simulink model "mpc_pathFollowingMod"  (R2024a)
settings: Solver=VariableStepAuto  StartTime=0.0  StopTime=10.0  RelTol=1e-3
PreLoadFcn:
  | load('pathFollowingUtil\pfcsubsystem_data.mat');
  | load('pathFollowingUtil\mpc_base.mat');
values from neighbouring files (symbols this model uses):
  Cf = evalin('base','Cf')    [helperSLTrajectoryFollowerWithRRScenarioSetup.m]
  Cr = evalin('base','Cr')    [helperSLTrajectoryFollowerWithRRScenarioSetup.m]
  Iz = evalin('base','Iz')    [helperSLTrajectoryFollowerWithRRScenarioSetup.m]
  lf = evalin('base','lf')    [helperSLTrajectoryFollowerWithRRScenarioSetup.m]
  lr = evalin('base','lr')    [helperSLTrajectoryFollowerWithRRScenarioSetup.m]
  m = worldActors(idx).actor_runtime.pose.matrix    [helperSLTrajectoryFollowerWithRRScenarioSetup.m]
  numReferencePose = 1    [HelperReferencePoseOnPath.m]
  pfcsubsystem_data =     [pfcsubsystem_data.mat]
undefined symbols (not defined in the file or in its folder): control_timeStep, DefaultSpacing, E_mpc, F_mpc, hasLag, InitialLongVel, NumEgoStates, sizeExNumSS, tau, tau2
libraries: mpcsigdimcheck_private x19, mpclib x3, simulink x2, sharedTrackingLibrary x1
(part 1 of 2)
settings Model: Creator=nobuakif  LastModifiedBy=fukuchi
settings DebuggingCC: UnderSpecifiedDimensionMsg=warning

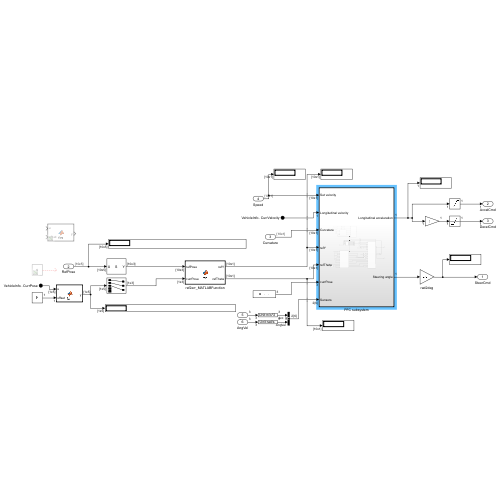
[thumbnail: Simulink's stored preview of the top-level diagram]
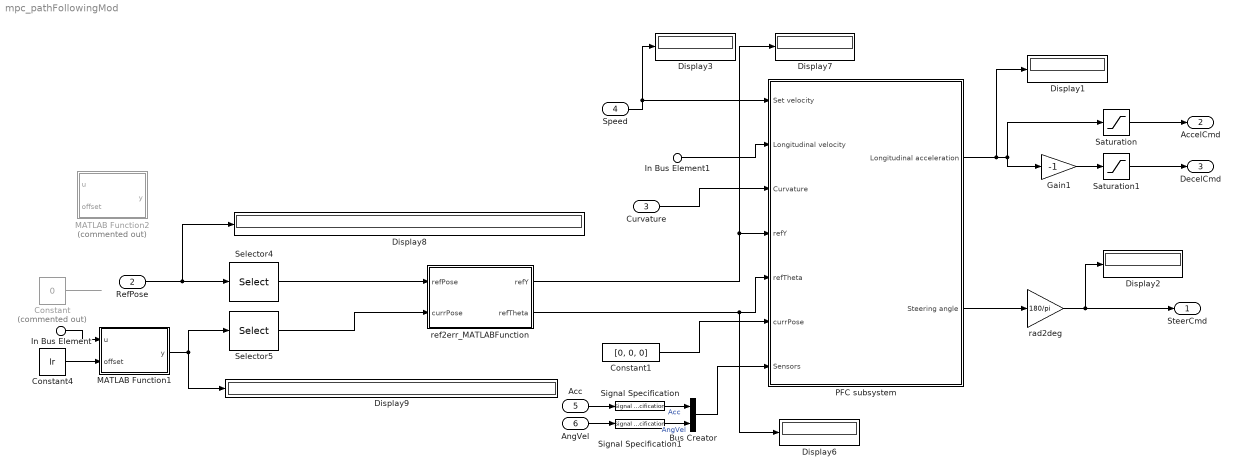
== system mpc_pathFollowingMod ==
  In Bus Element : Inport  PortName=VehicleInfo  Element=CurrPose
  In Bus Element1 : Inport  PortName=VehicleInfo  Element=CurrVelocity
  RefPose : Inport  Port=2  PortDimensions=[numReferencePose, 5]
  Curvature : Inport  Port=3  PortDimensions=[numReferencePose, 1]
  Speed : Inport  Port=4  PortDimensions=[numReferencePose, 1]
  Acc : Inport  Port=5  PortDimensions=3
  AngVel : Inport  Port=6  PortDimensions=3
  Bus Creator : BusCreator  Inputs=2
  Constant : Constant  Commented=on  Value=0
  Constant1 : Constant  Value=[0, 0, 0]
  Constant4 : Constant  Value=lr
  Display{1..3,6..9} (7 alike) : Display
  Gain1 : Gain  Gain=-1
  MATLAB Function1 : MATLAB Function  TreatAsAtomicUnit=on
  MATLAB Function2 : MATLAB Function  Commented=on  TreatAsAtomicUnit=on
  PFC subsystem : Subsystem  TreatAsAtomicUnit=on  VariantControl=Variant2
      settings: LibrarySourceBlock=mpclib/Automated Driving/Path Following Control System  RTWFileNameOpts=Use function name
  Saturation : Saturate  UpperLimit=inf  LowerLimit=0
  Saturation1 : Saturate  UpperLimit=inf  LowerLimit=0
  Selector4 : Selector  NumberOfDimensions=2  InputPortWidth=5  IndexOptions=Select all,Index vector (dialog)  Indices=[1:3],[1:3]  OutputSizes=1,1
  Selector5 : Selector  InputPortWidth=5  IndexOptions=Index vector (dialog)  Indices=[1:3]  OutputSizes=1
  Signal Specification : SignalSpecification  Unit=m/s^2
  Signal Specification1 : SignalSpecification  Unit=rad/s
  rad2deg : Gain  Gain=180/pi
  ref2err_MATLABFunction : MATLAB Function  TreatAsAtomicUnit=on
  SteerCmd : Outport
  AccelCmd : Outport  Port=2
  DecelCmd : Outport  Port=3
  wires:
  rad2deg/1 -> SteerCmd/1, Display2/1
  Saturation/1 -> AccelCmd/1
  Selector4/1 -> ref2err_MATLABFunction/1(refPose)
  Saturation1/1 -> DecelCmd/1
  MATLAB Function1/1(y) -> Selector5/1, Display9/1
  Selector5/1 -> ref2err_MATLABFunction/2(currPose)
  Constant/1 -> ?
  PFC subsystem/1(Longitudinal acceleration) -> Display1/1, Saturation/1, Gain1/1
  Constant4/1 -> MATLAB Function1/2(offset)
  In Bus Element/1 -> MATLAB Function1/1(u)
  RefPose/1 -> Display8/1, Selector4/1
  PFC subsystem/2(Steering angle) -> rad2deg/1
  In Bus Element1/1 -> PFC subsystem/2(Longitudinal velocity)
  Curvature/1 -> PFC subsystem/3(Curvature)
  ref2err_MATLABFunction/1(refY) -> PFC subsystem/4(refY), Display7/1
  ref2err_MATLABFunction/2(refTheta) -> Display6/1, PFC subsystem/5(refTheta)
  Speed/1 -> Display3/1, PFC subsystem/1(Set velocity)
  Gain1/1 -> Saturation1/1
  Constant1/1 -> PFC subsystem/6(currPose)
  Acc/1 -> Signal Specification/1
  Bus Creator/1 -> PFC subsystem/7(Sensors)
  AngVel/1 -> Signal Specification1/1
  Signal Specification/1 -> Bus Creator/1  "Acc"
  Signal Specification1/1 -> Bus Creator/2  "AngVel"

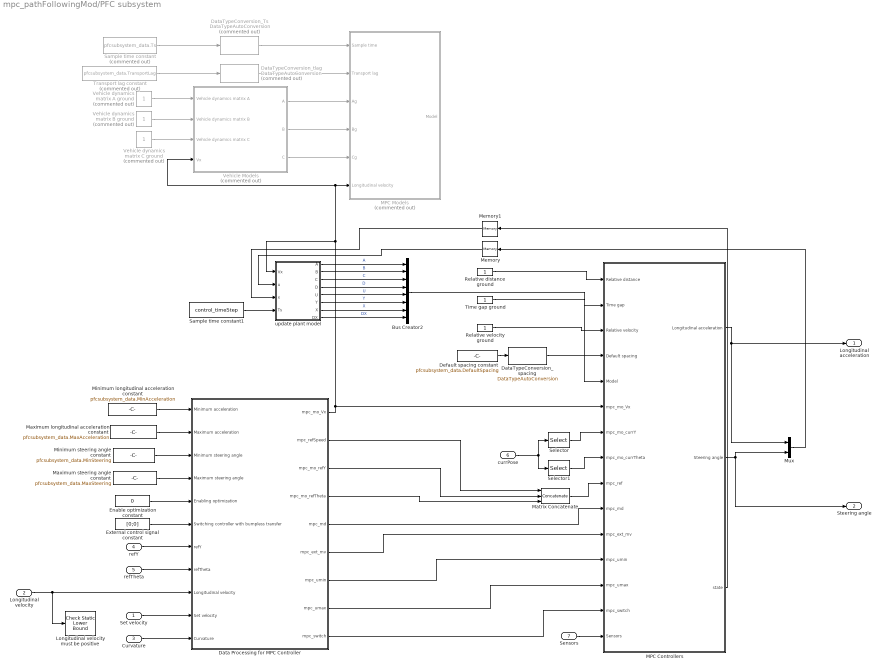
== system mpc_pathFollowingMod/PFC subsystem ==
  Set velocity : Inport
  Longitudinal velocity : Inport  Port=2
  Curvature : Inport  Port=3
  refY : Inport  Port=4
  refTheta : Inport  Port=5
  currPose : Inport  Port=6
  Sensors : Inport  Port=7
  Bus Creator2 : BusCreator  Inputs=8
  Data Processing for MPC Controller : Subsystem
  DataTypeConversion_Ts : mpcsigdimcheck_private/DataTypeAutoConversion  Commented=on  datatypestr=pfcsubsystem_data.DataType
  DataTypeConversion_spacing : mpcsigdimcheck_private/DataTypeAutoConversion  datatypestr=pfcsubsystem_data.DataType
  DataTypeConversion_tlag : mpcsigdimcheck_private/DataTypeAutoConversion  Commented=on  datatypestr=pfcsubsystem_data.DataType
  Default spacing constant : Constant  Value=pfcsubsystem_data.DefaultSpacing  OutDataTypeStr=pfcsubsystem_data.DataType
  Enable optimization constant : Constant  Value=0  OutDataTypeStr=pfcsubsystem_data.DataType
  External control signal constant : Constant  Value=[0;0]  VectorParams1D=off  OutDataTypeStr=pfcsubsystem_data.DataType
  Longitudinal velocity must be positive : simulink/Model Verification/Check Static  Lower Bound  Description=0 < u  min=0  min_included=off  enabled=on  stopWhenAssertionFail=on  export=off  icon=graphic
  MPC Controllers : Subsystem  Variant=on  VariantControlMode=label  VariantControl=Variant1  LabelModeActiveChoice=pathFollowingNoSpacingCtrl
  MPC Models : Subsystem  Commented=on  Variant=on  VariantControlMode=label  VariantControl=Variant1  LabelModeActiveChoice=pathFollowingNoSpacingCtrl
  Matrix Concatenate : Concatenate  NumInputs=3  Mode=Multidimensional array  ConcatenateDimension=2
  Maximum longitudinal acceleration constant : Constant  Value=pfcsubsystem_data.MaxAcceleration  OutDataTypeStr=pfcsubsystem_data.DataType
  Maximum steering angle constant : Constant  Value=pfcsubsystem_data.MaxSteering  OutDataTypeStr=pfcsubsystem_data.DataType
  Memory : Memory
  Memory1 : Memory
  Minimum longitudinal acceleration constant : Constant  Value=pfcsubsystem_data.MinAcceleration  OutDataTypeStr=pfcsubsystem_data.DataType
  Minimum steering angle constant : Constant  Value=pfcsubsystem_data.MinSteering  OutDataTypeStr=pfcsubsystem_data.DataType
  Mux : Mux  Inputs=2
  Relative distance ground : Constant  OutDataTypeStr=pfcsubsystem_data.DataType
  Relative velocity ground : Constant  OutDataTypeStr=pfcsubsystem_data.DataType
  Sample time constant : Constant  Commented=on  Value=pfcsubsystem_data.Ts  OutDataTypeStr=pfcsubsystem_data.DataType
  Sample time constant1 : Constant  Value=control_timeStep  OutDataTypeStr=pfcsubsystem_data.DataType
  Selector : Selector  InputPortWidth=3  IndexOptions=Index vector (dialog)  Indices=2  OutputSizes=1
  Selector1 : Selector  InputPortWidth=3  IndexOptions=Index vector (dialog)  Indices=3  OutputSizes=1
  Time gap ground : Constant  OutDataTypeStr=pfcsubsystem_data.DataType
  Transport lag constant : Constant  Commented=on  Value=pfcsubsystem_data.TransportLag  OutDataTypeStr=pfcsubsystem_data.DataType
  Vehicle Models : Subsystem  Commented=on  Variant=on  VariantControlMode=label  VariantControl=Variant1  LabelModeActiveChoice=useVehicleParameters
  Vehicle dynamics matrix A ground : Constant  Commented=on  OutDataTypeStr=pfcsubsystem_data.DataType
  Vehicle dynamics matrix B ground : Constant  Commented=on  OutDataTypeStr=pfcsubsystem_data.DataType
  Vehicle dynamics matrix C ground : Constant  Commented=on  OutDataTypeStr=pfcsubsystem_data.DataType
  update plant model : MATLAB Function  TreatAsAtomicUnit=on
  Longitudinal acceleration : Outport  PortDimensions=1  VectorParamsAs1DForOutWhenUnconnected=off
  Steering angle : Outport  Port=2  VectorParamsAs1DForOutWhenUnconnected=off
  wires:
  Relative velocity ground/1 -> MPC Controllers/3("Relative velocity ")
  Relative distance ground/1 -> MPC Controllers/1("Relative distance ")
  Time gap ground/1 -> MPC Controllers/2("Time gap ")
  MPC Controllers/1(" Longitudinal acceleration") -> Longitudinal acceleration/1, Mux/1
  Default spacing constant/1 -> DataTypeConversion_spacing/1
  Data Processing for MPC Controller/9(mpc_switch) -> MPC Controllers/14("mpc_switch ")
  Bus Creator2/1 -> MPC Controllers/5("Model ")
  Data Processing for MPC Controller/8(mpc_umax) -> MPC Controllers/13("mpc_umax ")
  Data Processing for MPC Controller/1(mpc_mo_Vx) -> update plant model/1(Vx), MPC Models/6("Longitudinal velocity "), Vehicle Models/4("Vx "), MPC Controllers/6("mpc_mo_Vx ")
  Data Processing for MPC Controller/5(mpc_md) -> MPC Controllers/10("mpc_md ")
  Data Processing for MPC Controller/4(mpc_mo_refTheta) -> Matrix Concatenate/3
  Data Processing for MPC Controller/2(mpc_refSpeed) -> Matrix Concatenate/1
  Longitudinal velocity/1 -> Data Processing for MPC Controller/9(Longitudinal velocity), Longitudinal velocity must be positive/1
  Data Processing for MPC Controller/3(mpc_mo_refY) -> Matrix Concatenate/2
  Data Processing for MPC Controller/6(mpc_ext_mv) -> MPC Controllers/11("mpc_ext_mv ")
  Data Processing for MPC Controller/7(mpc_umin) -> MPC Controllers/12("mpc_umin ")
  Curvature/1 -> Data Processing for MPC Controller/11(Curvature)
  Set velocity/1 -> Data Processing for MPC Controller/10(Set velocity)
  refY/1 -> Data Processing for MPC Controller/7(refY)
  refTheta/1 -> Data Processing for MPC Controller/8(refTheta)
  Maximum longitudinal acceleration constant/1 -> Data Processing for MPC Controller/2(Maximum acceleration)
  Maximum steering angle constant/1 -> Data Processing for MPC Controller/4(Maximum steering angle)
  Enable optimization constant/1 -> Data Processing for MPC Controller/5(Enabling optimization)
  External control signal constant/1 -> Data Processing for MPC Controller/6(Switching controller with bumpless transfer)
  Minimum longitudinal acceleration constant/1 -> Data Processing for MPC Controller/1(Minimum acceleration)
  Minimum steering angle constant/1 -> Data Processing for MPC Controller/3(Minimum steering angle)
  Vehicle Models/1(" A") -> MPC Models/3(Ag)
  Vehicle Models/2(" B") -> MPC Models/4(Bg)
  Vehicle Models/3(" C") -> MPC Models/5(Cg)
  Transport lag constant/1 -> DataTypeConversion_tlag/1
  Sample time constant/1 -> DataTypeConversion_Ts/1
  Vehicle dynamics matrix A ground/1 -> Vehicle Models/1(Vehicle dynamics matrix A)
  Vehicle dynamics matrix C ground/1 -> Vehicle Models/3(Vehicle dynamics matrix C)
  Vehicle dynamics matrix B ground/1 -> Vehicle Models/2(Vehicle dynamics matrix B)
  DataTypeConversion_Ts/1 -> MPC Models/1(Sample time)
  DataTypeConversion_tlag/1 -> MPC Models/2(Transport lag)
  DataTypeConversion_spacing/1 -> MPC Controllers/4("Default spacing ")
  Sample time constant1/1 -> update plant model/4(Ts)
  update plant model/1(A) -> Bus Creator2/1  "A"
  update plant model/2(B) -> Bus Creator2/2  "B"
  update plant model/3(C) -> Bus Creator2/3  "C"
  update plant model/4(D) -> Bus Creator2/4  "D"
  update plant model/5(U) -> Bus Creator2/5  "U"
  update plant model/6(Y) -> Bus Creator2/6  "Y"
  update plant model/7(X) -> Bus Creator2/7  "X"
  update plant model/8(DX) -> Bus Creator2/8  "DX"
  Mux/1 -> Memory/1
  MPC Controllers/3(state) -> Memory1/1
  Memory/1 -> update plant model/2(u)
  Matrix Concatenate/1 -> MPC Controllers/9("mpc_ref ")
  Selector/1 -> MPC Controllers/7(mpc_mo_currY)
  Selector1/1 -> MPC Controllers/8(mpc_mo_currTheta)
  currPose/1 -> Selector1/1, Selector/1
  Memory1/1 -> update plant model/3(x)
  MPC Controllers/2("  Steering angle") -> Mux/2, Steering angle/1
  Sensors/1 -> MPC Controllers/15(Sensors)

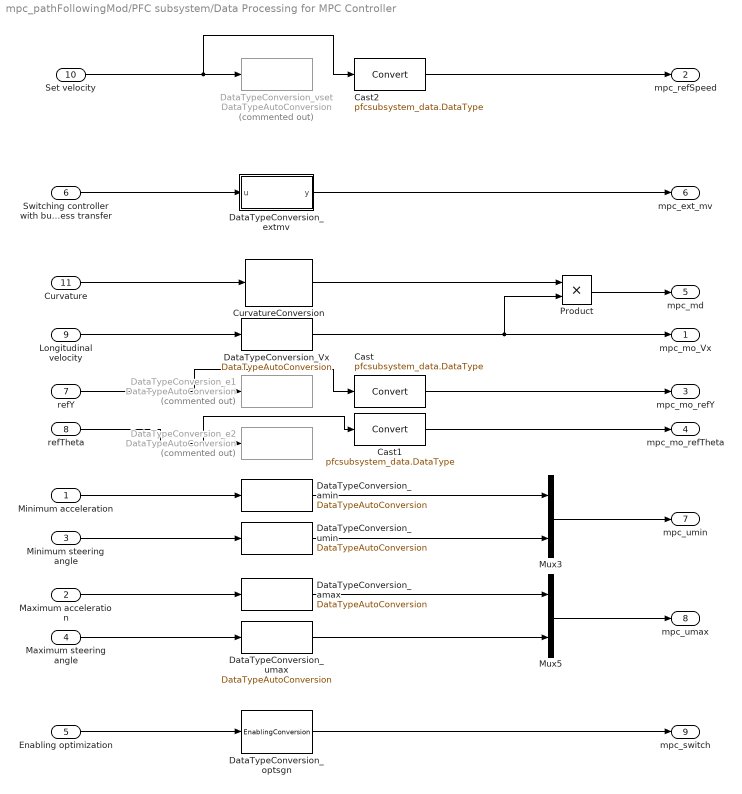
== system mpc_pathFollowingMod/PFC subsystem/Data Processing for MPC Controller ==
  Minimum acceleration : Inport
  Maximum acceleration : Inport  Port=2
  Minimum steering angle : Inport  Port=3
  Maximum steering angle : Inport  Port=4
  Enabling optimization : Inport  Port=5
  Switching controller with bumpless transfer : Inport  Port=6
  refY : Inport  Port=7
  refTheta : Inport  Port=8
  Longitudinal velocity : Inport  Port=9
  Set velocity : Inport  Port=10
  Curvature : Inport  Port=11
  Cast : DataTypeConversion  OutDataTypeStr=pfcsubsystem_data.DataType  SaturateOnIntegerOverflow=off  RndMeth=Floor
  Cast1 : DataTypeConversion  OutDataTypeStr=pfcsubsystem_data.DataType  SaturateOnIntegerOverflow=off  RndMeth=Floor
  Cast2 : DataTypeConversion  OutDataTypeStr=pfcsubsystem_data.DataType  SaturateOnIntegerOverflow=off  RndMeth=Floor
  CurvatureConversion : mpcsigdimcheck_private/CurvatureConversion  datatypestr=pfcsubsystem_data.DataType  p=pfcsubsystem_data.Controller.PredictionHorizon
  DataTypeConversion_Vx : mpcsigdimcheck_private/DataTypeAutoConversion  datatypestr=pfcsubsystem_data.DataType
  DataTypeConversion_amax : mpcsigdimcheck_private/DataTypeAutoConversion  datatypestr=pfcsubsystem_data.DataType
  DataTypeConversion_amin : mpcsigdimcheck_private/DataTypeAutoConversion  datatypestr=pfcsubsystem_data.DataType
  DataTypeConversion_e1 : mpcsigdimcheck_private/DataTypeAutoConversion  Commented=on  datatypestr=pfcsubsystem_data.DataType
  DataTypeConversion_e2 : mpcsigdimcheck_private/DataTypeAutoConversion  Commented=on  datatypestr=pfcsubsystem_data.DataType
  DataTypeConversion_extmv : MATLAB Function  TreatAsAtomicUnit=on  mask(MPCDataTypeAutoConversion){datatypestr=pfcsubsystem_data.DataType}
      mask prompts: datatypestr "Data type"
      mask init:
      | isDouble = strcmp(datatypestr,'double');
  DataTypeConversion_optsgn : mpcsigdimcheck_private/EnablingConversion  SystemSampleTime=-1  VariantActivationTime=update diagram  AllowFlexibleInterface=on  Latency=0  AutoFrameSizeCalculation=off
  DataTypeConversion_umax : mpcsigdimcheck_private/DataTypeAutoConversion  datatypestr=pfcsubsystem_data.DataType
  DataTypeConversion_umin : mpcsigdimcheck_private/DataTypeAutoConversion  datatypestr=pfcsubsystem_data.DataType
  DataTypeConversion_vset : mpcsigdimcheck_private/DataTypeAutoConversion  Commented=on  datatypestr=pfcsubsystem_data.DataType
  Mux3 : Mux  Inputs=2
  Mux5 : Mux  Inputs=2
  Product : Product
  mpc_mo_Vx : Outport  VectorParamsAs1DForOutWhenUnconnected=off
  mpc_refSpeed : Outport  Port=2  VectorParamsAs1DForOutWhenUnconnected=off
  mpc_mo_refY : Outport  Port=3  VectorParamsAs1DForOutWhenUnconnected=off
  mpc_mo_refTheta : Outport  Port=4  VectorParamsAs1DForOutWhenUnconnected=off
  mpc_md : Outport  Port=5  VectorParamsAs1DForOutWhenUnconnected=off
  mpc_ext_mv : Outport  Port=6  VectorParamsAs1DForOutWhenUnconnected=off
  mpc_umin : Outport  Port=7  VectorParamsAs1DForOutWhenUnconnected=off
  mpc_umax : Outport  Port=8  VectorParamsAs1DForOutWhenUnconnected=off
  mpc_switch : Outport  Port=9  VectorParamsAs1DForOutWhenUnconnected=off
  wires:
  Longitudinal velocity/1 -> DataTypeConversion_Vx/1
  Curvature/1 -> CurvatureConversion/1
  Mux5/1 -> mpc_umax/1
  Maximum steering angle/1 -> DataTypeConversion_umax/1
  Minimum steering angle/1 -> DataTypeConversion_umin/1
  DataTypeConversion_amin/1 -> Mux3/1
  CurvatureConversion/1 -> Product/1
  Product/1 -> mpc_md/1
  refTheta/1 -> Cast1/1, DataTypeConversion_e2/1
  Maximum acceleration/1 -> DataTypeConversion_amax/1
  refY/1 -> Cast/1, DataTypeConversion_e1/1
  DataTypeConversion_umin/1 -> Mux3/2
  DataTypeConversion_amax/1 -> Mux5/1
  DataTypeConversion_Vx/1 -> mpc_mo_Vx/1, Product/2
  DataTypeConversion_umax/1 -> Mux5/2
  Minimum acceleration/1 -> DataTypeConversion_amin/1
  Switching controller with bumpless transfer/1 -> DataTypeConversion_extmv/1(u)
  DataTypeConversion_extmv/1(y) -> mpc_ext_mv/1
  Mux3/1 -> mpc_umin/1
  Set velocity/1 -> Cast2/1, DataTypeConversion_vset/1
  Cast/1 -> mpc_mo_refY/1
  Enabling optimization/1 -> DataTypeConversion_optsgn/1
  DataTypeConversion_optsgn/1 -> mpc_switch/1
  Cast1/1 -> mpc_mo_refTheta/1
  Cast2/1 -> mpc_refSpeed/1

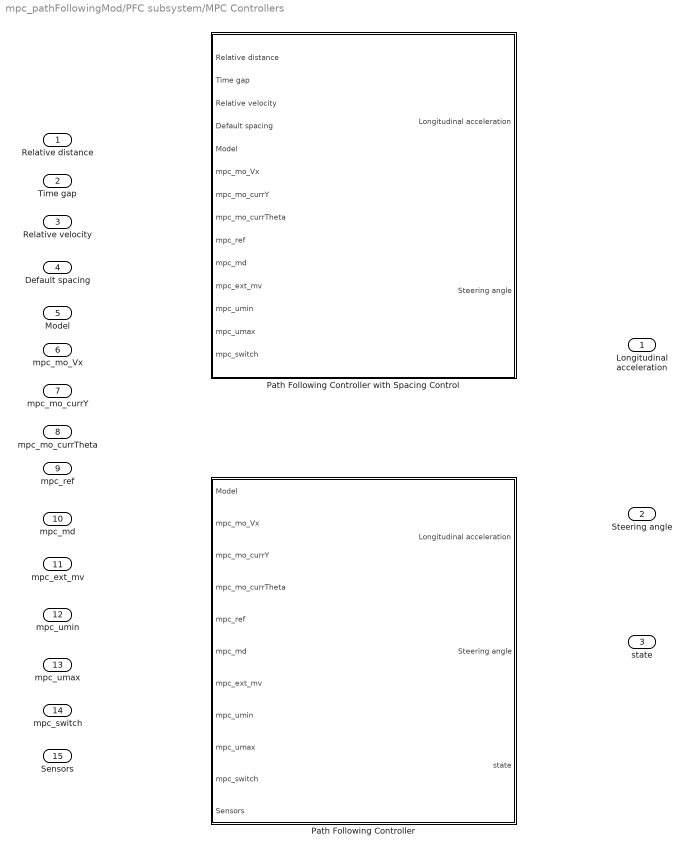
== system mpc_pathFollowingMod/PFC subsystem/MPC Controllers ==
  "Relative distance " : Inport
  "Time gap " : Inport  Port=2
  "Relative velocity " : Inport  Port=3
  "Default spacing " : Inport  Port=4
  "Model " : Inport  Port=5
  "mpc_mo_Vx " : Inport  Port=6
  mpc_mo_currY : Inport  Port=7
  mpc_mo_currTheta : Inport  Port=8
  "mpc_ref " : Inport  Port=9
  "mpc_md " : Inport  Port=10
  "mpc_ext_mv " : Inport  Port=11
  "mpc_umin " : Inport  Port=12
  "mpc_umax " : Inport  Port=13
  "mpc_switch " : Inport  Port=14
  Sensors : Inport  Port=15
  Path Following Controller : Subsystem  VariantControl=pathFollowingNoSpacingCtrl
  Path Following Controller with Spacing Control : Subsystem  VariantControl=pathFollowingHasSpacingCtrl
  " Longitudinal acceleration" : Outport  VectorParamsAs1DForOutWhenUnconnected=off
  "  Steering angle" : Outport  Port=2  VectorParamsAs1DForOutWhenUnconnected=off
  state : Outport  Port=3

== system mpc_pathFollowingMod/PFC subsystem/MPC Models ==
  Sample time : Inport
  Transport lag : Inport  Port=2
  Ag : Inport  Port=3
  Bg : Inport  Port=4
  Cg : Inport  Port=5
  "Longitudinal velocity " : Inport  Port=6
  MPC Model : Subsystem  VariantControl=pathFollowingNoSpacingCtrl
  MPC Model with Spacing Control : Subsystem  VariantControl=pathFollowingHasSpacingCtrl
  " Model" : Outport  VectorParamsAs1DForOutWhenUnconnected=off

== system mpc_pathFollowingMod/PFC subsystem/Vehicle Models ==
  Vehicle dynamics matrix A : Inport
  Vehicle dynamics matrix B : Inport  Port=2
  Vehicle dynamics matrix C : Inport  Port=3
  "Vx " : Inport  Port=4
  Vehicle external model : Subsystem  VariantControl=useVehicleModel
  Vehicle parametric model : Subsystem  VariantControl=useVehicleParameters
  " A" : Outport  VectorParamsAs1DForOutWhenUnconnected=off
  " B" : Outport  Port=2  VectorParamsAs1DForOutWhenUnconnected=off
  " C" : Outport  Port=3  VectorParamsAs1DForOutWhenUnconnected=off

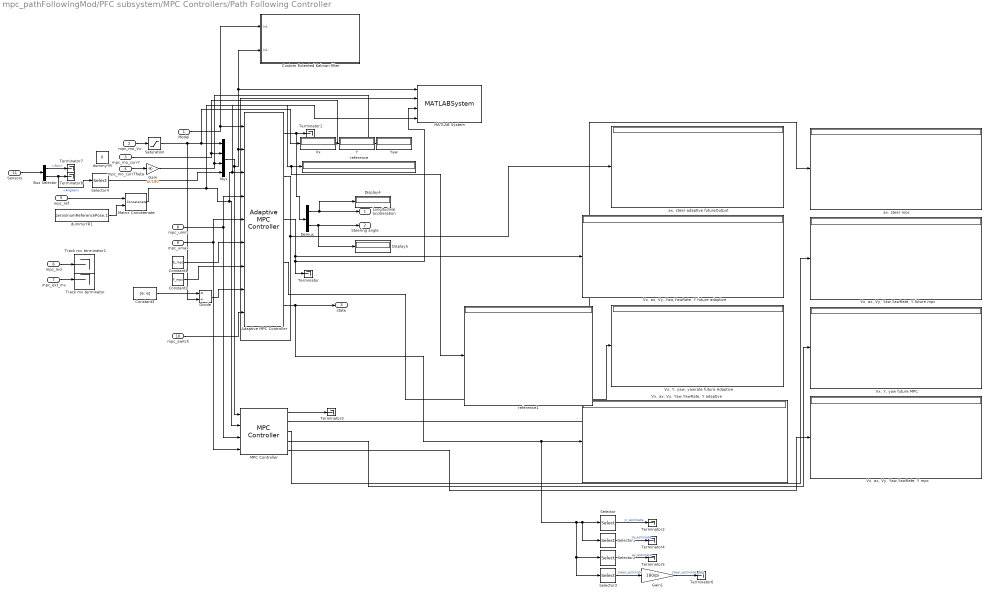
== system mpc_pathFollowingMod/PFC subsystem/MPC Controllers/Path Following Controller ==
  Model : Inport
  mpc_mo_Vx : Inport  Port=2
  mpc_mo_currY : Inport  Port=3
  mpc_mo_currTheta : Inport  Port=4
  mpc_ref : Inport  Port=5
  mpc_md : Inport  Port=6
  mpc_ext_mv : Inport  Port=7
  mpc_umin : Inport  Port=8
  mpc_umax : Inport  Port=9
  mpc_switch : Inport  Port=10
  Sensors : Inport  Port=11
  Adaptive MPC Controller : mpclib/Adaptive MPC Controller  SCDEnableBlockLinearizationSpecification=on  mpcobj=mpc_base  x0=state_init  enable_value=0  updateMPCinCallerWorkspace=off  md_inport=off  mv_inport=off  uref_inport=off  return_cost=off  return_mvseq=on  return_qpstatus=off  return_xseq=on  return_state=on  return_ovseq=on  state_inport=off  isltv_plant=off  umin_inport=on  umax_inport=on  ymin_inport=off  ymax_inport=off  cc_inport=on  ywt_inport=off  uwt_inport=off  duwt_inport=off  rhoeps_inport=off  pm_inport=off  MaximumP=10  HorizonChoice=FixedHorizon  BlockDataType=double  SampleTimeInherited=on  switch_inport=on
  Bus Selector : BusSelector  OutputSignals=Acc,AngVel
  Constant1 : Constant  Value=E_mpc
  Constant2 : Constant  Value=F_mpc
  Constant3 : Constant  Value=[6; 6]
  Custom Extented Kalman filter : Subsystem
  Demux : Demux  Outputs=2
  Display4 : Display
  Display5 : Display
  Divide : Product  Inputs=*/
  Gain : Gain  Gain=pi/180
  Gain1 : Gain  Gain=180/pi
  MATLAB System : MATLABSystem  System=MPCVisualizer  PredictionHorizon=numReferencePose  SampleTime=control_timeStep  VideoFlag=off  VideoFileName=mpc_visualization.mp4  stateoffset=sizeExNumSS  YLimVx=[0, 25]  YLimY=[-10, 10]  YLimYaw=[-pi/6, pi/6]  YLimYawRate=[-pi/6, pi/6]  YLimSteer=[-pi/6, pi/6]  YLimAx=[-10, 2]  YLimVy=[-2, 2]
      mask Type: MPCVisualizer
      mask Display:
      | disp('MPCVisualizer');
      | port_label('input',1,'measured');
      | port_label('input',2,'manipulated');
      | port_label('input',3,'state');
      | port_label('input',4,'reference');
  MPC Controller : mpclib/MPC Controller  SCDEnableBlockLinearizationSpecification=on  mpcobj=mpc_base  x0=state_init  is_multiple=0  enable_value=0  return_u0=off  updateMPCinCallerWorkspace=on  md_inport=off  mv_inport=off  uref_inport=off  return_cost=off  return_mvseq=on  return_qpstatus=off  return_xseq=on  return_state=on  return_ovseq=on  state_inport=off  umin_inport=on  umax_inport=on  ymin_inport=off  ymax_inport=off  cc_inport=off  ywt_inport=off  uwt_inport=off  duwt_inport=off  rhoeps_inport=off  pm_inport=off  MaximumP=10  HorizonChoice=FixedHorizon  n_ts=0.1  n_p=10  n_mv=2  n_md=0  n_ud=0  n_mo=4  n_uo=0  BlockDataType=double  SampleTimeInherited=off  switch_inport=off
  Matrix Concatenate : Concatenate  Mode=Multidimensional array  ConcatenateDimension=2
  Mux : Mux
  Saturation : Saturate  UpperLimit=inf  LowerLimit=eps
  Selector : Selector  InputPortWidth=6+sizeExNumSS  IndexOptions=Index vector (dialog)  Indices=5+sizeExNumSS  OutputSizes=1
  Selector1 : Selector  InputPortWidth=6+sizeExNumSS  IndexOptions=Index vector (dialog)  Indices=5+sizeExNumSS  OutputSizes=1
  Selector2 : Selector  InputPortWidth=6+sizeExNumSS  IndexOptions=Index vector (dialog)  Indices=2+sizeExNumSS  OutputSizes=1
  Selector3 : Selector  InputPortWidth=6+sizeExNumSS  IndexOptions=Index vector (dialog)  Indices=1  OutputSizes=1
  Selector4 : Selector  InputPortWidth=3  IndexOptions=Index vector (dialog)  Indices=3  OutputSizes=1
  Terminator{,1..8} (9 alike) : Terminator
  Track mv terminator : Terminator
  Track mv terminator1 : Terminator
  Vx : Display
  "Vx, Y, yaw future MPC" : Display
  "Vx, Y, yaw, yawrate future Adaptive" : Display
  "Vx, ax, Vy, Yaw,YawRate, Y adaptive" : Display
  "Vx, ax, Vy, Yaw,YawRate, Y future adaptive" : Display
  "Vx, ax, Vy, Yaw,YawRate, Y future mpc" : Display
  "Vx, ax, Vy, Yaw,YawRate, Y mpc" : Display
  Y : Display
  Yaw : Display
  "ax, steer adaptive futureOutput" : Display
  "ax, steer mpc" : Display
  dummyYR : Constant  Value=0
  dummyYR1 : Constant  Value=zeros(numReferencePose,1)
  reference : Display
  reference1 : Display
  Longitudinal acceleration : Outport  Unit=m/s^2  VectorParamsAs1DForOutWhenUnconnected=off
  " Steering angle" : Outport  Port=2  Unit=rad  VectorParamsAs1DForOutWhenUnconnected=off
  state : Outport  Port=3
  wires:
  mpc_mo_Vx/1 -> Saturation/1
  Adaptive MPC Controller/1 -> Demux/1, Terminator1/1
  Mux/1 -> MPC Controller/1, Custom Extented Kalman filter/2(In2), MATLAB System/1, Adaptive MPC Controller/2
  Model/1 -> Custom Extented Kalman filter/1(In1), Adaptive MPC Controller/1
  mpc_mo_currTheta/1 -> Gain/1
  Matrix Concatenate/1 -> reference1/1, reference/1, MATLAB System/4, Adaptive MPC Controller/3, MPC Controller/2
  mpc_md/1 -> Track mv terminator1/1
  mpc_umax/1 -> MPC Controller/4, Adaptive MPC Controller/5
  mpc_umin/1 -> MPC Controller/3, Adaptive MPC Controller/4
  mpc_switch/1 -> Adaptive MPC Controller/9
  Demux/1 -> Display4/1, Longitudinal acceleration/1
  mpc_ext_mv/1 -> Track mv terminator/1
  Adaptive MPC Controller/3 -> MATLAB System/3, Terminator/1, "Vx, ax, Vy, Yaw,YawRate, Y future adaptive"/1
  Adaptive MPC Controller/4 -> "Vx, Y, yaw, yawrate future Adaptive"/1
  Adaptive MPC Controller/2 -> MATLAB System/2, "ax, steer adaptive futureOutput"/1
  MPC Controller/1 -> Terminator3/1
  MPC Controller/2 -> "ax, steer mpc"/1
  MPC Controller/3 -> "Vx, ax, Vy, Yaw,YawRate, Y future mpc"/1
  MPC Controller/4 -> "Vx, Y, yaw future MPC"/1
  MPC Controller/5 -> "Vx, ax, Vy, Yaw,YawRate, Y mpc"/1
  Adaptive MPC Controller/5 -> state/1, Selector3/1, Selector2/1, Selector1/1, Selector/1, "Vx, ax, Vy, Yaw,YawRate, Y adaptive"/1
  Demux/2 -> " Steering angle"/1, Display5/1
  Selector4/1 -> Mux/4
  mpc_ref/1 -> Matrix Concatenate/1
  dummyYR1/1 -> Matrix Concatenate/2
  Constant1/1 -> Adaptive MPC Controller/6
  Constant2/1 -> Adaptive MPC Controller/7
  Constant3/1 -> Divide/1
  Divide/1 -> Adaptive MPC Controller/8
  Saturation/1 -> Vx/1, Mux/1, Divide/2
  Selector/1 -> Terminator2/1  "yr_estimate"
  Selector1/1 -> Terminator4/1  "Vy_estimate"
  Selector2/1 -> Terminator5/1  "ax_estimate"
  Selector3/1 -> Gain1/1  "steer_estimate"
  Sensors/1 -> Bus Selector/1
  Bus Selector/1 -> Terminator7/1  "<Acc>"
  Bus Selector/2 -> Selector4/1, Terminator8/1  "<AngVel>"
  Gain1/1 -> Terminator6/1  "steer_estimate_deg"
  mpc_mo_currY/1 -> Y/1, Mux/2
  Gain/1 -> Yaw/1, Mux/3

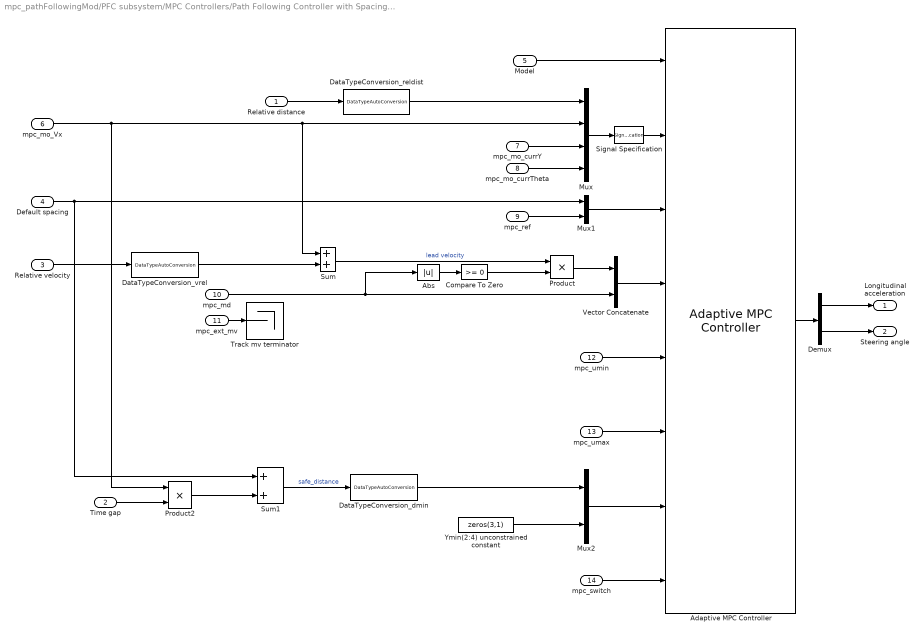
== system mpc_pathFollowingMod/PFC subsystem/MPC Controllers/Path Following Controller with Spacing Control ==
  Relative distance : Inport  Unit=m
  Time gap : Inport  Port=2
  Relative velocity : Inport  Port=3  Unit=m/s
  Default spacing : Inport  Port=4
  Model : Inport  Port=5
  mpc_mo_Vx : Inport  Port=6
  mpc_mo_currY : Inport  Port=7
  mpc_mo_currTheta : Inport  Port=8
  mpc_ref : Inport  Port=9
  mpc_md : Inport  Port=10
  mpc_ext_mv : Inport  Port=11
  mpc_umin : Inport  Port=12
  mpc_umax : Inport  Port=13
  mpc_switch : Inport  Port=14
  Abs : Abs  ZeroCross=off  SaturateOnIntegerOverflow=off
  Adaptive MPC Controller : mpclib/Adaptive MPC Controller  SCDEnableBlockLinearizationSpecification=on  mpcobj=mpcobj  enable_value=0  updateMPCinCallerWorkspace=off  md_inport=on  mv_inport=off  uref_inport=off  return_cost=off  return_mvseq=off  return_qpstatus=off  return_xseq=off  return_state=off  return_ovseq=off  state_inport=off  isltv_plant=off  umin_inport=on  umax_inport=on  ymin_inport=on  ymax_inport=off  cc_inport=off  ywt_inport=off  uwt_inport=off  duwt_inport=off  rhoeps_inport=off  pm_inport=off  MaximumP=10  HorizonChoice=FixedHorizon  BlockDataType=double  SampleTimeInherited=off  switch_inport=on
  Compare To Zero : simulink/Logic and Bit Operations/Compare To Zero  relop=>=  OutDataTypeStr=boolean  ZeroCross=off
  DataTypeConversion_dmin : mpcsigdimcheck_private/DataTypeAutoConversion  datatypestr=pfcsubsystem_data.DataType
  DataTypeConversion_reldist : mpcsigdimcheck_private/DataTypeAutoConversion  datatypestr=pfcsubsystem_data.DataType
  DataTypeConversion_vrel : mpcsigdimcheck_private/DataTypeAutoConversion  datatypestr=pfcsubsystem_data.DataType
  Demux : Demux  Outputs=2
  Mux : Mux
  Mux1 : Mux  Inputs=2
  Mux2 : Mux  Inputs=2
  Product : Product
  Product2 : Product
  Signal Specification : SignalSpecification  Dimensions=4
  Sum : Sum
  Sum1 : Sum
  Track mv terminator : Terminator
  Vector Concatenate : Concatenate  Mode=Multidimensional array  ConcatenateDimension=2
  Ymin(2:4) unconstrained constant : Constant  Value=zeros(3,1)  VectorParams1D=off  OutDataTypeStr=pfcsubsystem_data.DataType
  Longitudinal acceleration : Outport  Unit=m/s^2  VectorParamsAs1DForOutWhenUnconnected=off
  " Steering angle" : Outport  Port=2  Unit=rad  VectorParamsAs1DForOutWhenUnconnected=off
  wires:
  Mux2/1 -> Adaptive MPC Controller/7
  Ymin(2:4) unconstrained constant/1 -> Mux2/2
  DataTypeConversion_reldist/1 -> Mux/1
  mpc_umin/1 -> Adaptive MPC Controller/5
  Demux/1 -> Longitudinal acceleration/1
  Model/1 -> Adaptive MPC Controller/1
  mpc_mo_currTheta/1 -> Mux/4
  Mux/1 -> Signal Specification/1
  Default spacing/1 -> Mux1/1, Sum1/1
  Relative velocity/1 -> DataTypeConversion_vrel/1
  mpc_mo_Vx/1 -> Product2/1, Mux/2, Sum/1
  mpc_umax/1 -> Adaptive MPC Controller/6
  Mux1/1 -> Adaptive MPC Controller/3
  Relative distance/1 -> DataTypeConversion_reldist/1
  Product2/1 -> Sum1/2
  mpc_switch/1 -> Adaptive MPC Controller/8
  Adaptive MPC Controller/1 -> Demux/1
  mpc_mo_currY/1 -> Mux/3
  Time gap/1 -> Product2/2
  Sum1/1 -> DataTypeConversion_dmin/1  "safe_distance"
  Sum/1 -> Product/1  "lead velocity"
  Demux/2 -> " Steering angle"/1
  DataTypeConversion_dmin/1 -> Mux2/1
  Signal Specification/1 -> Adaptive MPC Controller/2
  Vector Concatenate/1 -> Adaptive MPC Controller/4
  mpc_ref/1 -> Mux1/2
  mpc_ext_mv/1 -> Track mv terminator/1
  DataTypeConversion_vrel/1 -> Sum/2
  Abs/1 -> Compare To Zero/1
  mpc_md/1 -> Abs/1, Vector Concatenate/2
  Compare To Zero/1 -> Product/2
  Product/1 -> Vector Concatenate/1

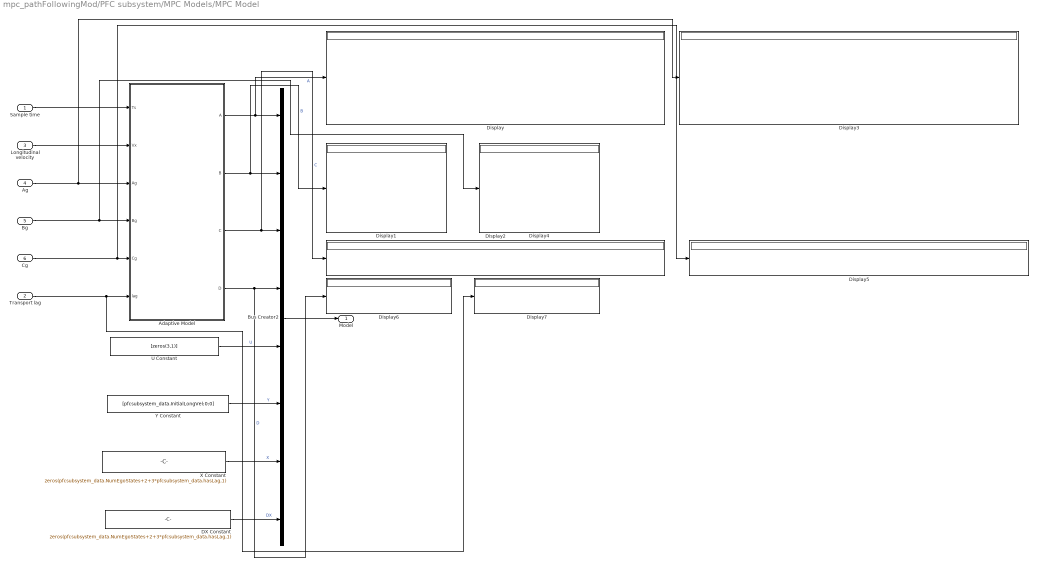
== system mpc_pathFollowingMod/PFC subsystem/MPC Models/MPC Model ==
  Sample time : Inport
  Transport lag : Inport  Port=2
  Longitudinal velocity : Inport  Port=3
  Ag : Inport  Port=4
  Bg : Inport  Port=5
  Cg : Inport  Port=6
  Adaptive Model : MATLAB Function  TreatAsAtomicUnit=on
  Bus Creator2 : BusCreator  Inputs=8
  DX Constant : Constant  Value=zeros(pfcsubsystem_data.NumEgoStates+2+3*pfcsubsystem_data.hasLag,1)  VectorParams1D=off  OutDataTypeStr=pfcsubsystem_data.DataType
  Display{,1..7} (8 alike) : Display
  U Constant : Constant  Value=[zeros(3,1)]  VectorParams1D=off  OutDataTypeStr=pfcsubsystem_data.DataType
  X Constant : Constant  Value=zeros(pfcsubsystem_data.NumEgoStates+2+3*pfcsubsystem_data.hasLag,1)  VectorParams1D=off  OutDataTypeStr=pfcsubsystem_data.DataType
  Y Constant : Constant  Value=[pfcsubsystem_data.InitialLongVel;0;0]  VectorParams1D=off  OutDataTypeStr=pfcsubsystem_data.DataType
  Model : Outport  VectorParamsAs1DForOutWhenUnconnected=off
  wires:
  Adaptive Model/2(B) -> Display1/1, Bus Creator2/2  "B"
  Transport lag/1 -> Display7/1, Adaptive Model/6(lag)
  U Constant/1 -> Bus Creator2/5  "U"
  DX Constant/1 -> Bus Creator2/8  "DX"
  Adaptive Model/3(C) -> Display2/1, Bus Creator2/3  "C"
  Adaptive Model/4(D) -> Display6/1, Bus Creator2/4  "D"
  Longitudinal velocity/1 -> Adaptive Model/2(Vx)
  Adaptive Model/1(A) -> Display/1, Bus Creator2/1  "A"
  Sample time/1 -> Adaptive Model/1(Ts)
  Y Constant/1 -> Bus Creator2/6  "Y"
  X Constant/1 -> Bus Creator2/7  "X"
  Bus Creator2/1 -> Model/1
  Ag/1 -> Display3/1, Adaptive Model/3(Ag)
  Bg/1 -> Display4/1, Adaptive Model/4(Bg)
  Cg/1 -> Display5/1, Adaptive Model/5(Cg)

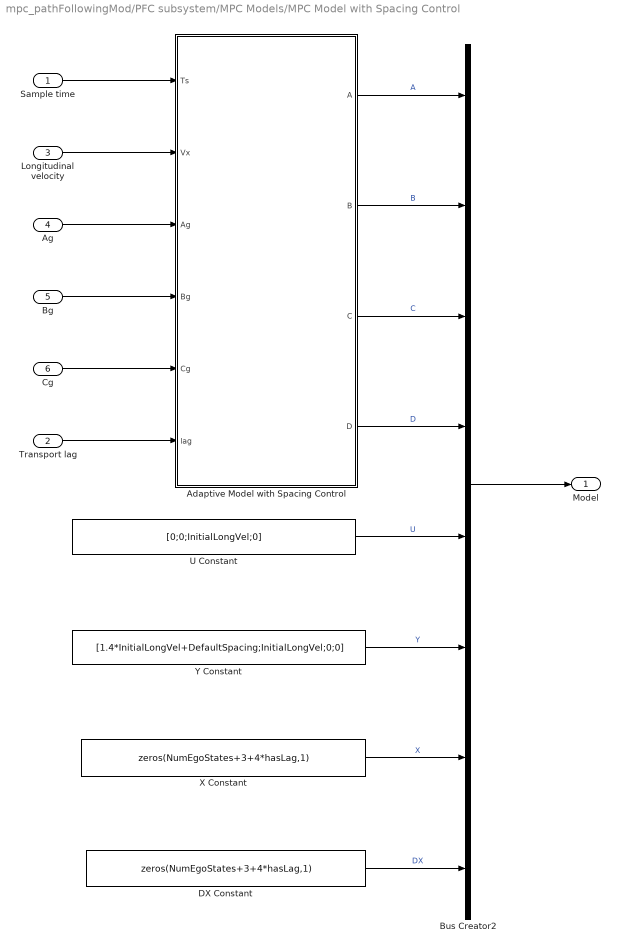
== system mpc_pathFollowingMod/PFC subsystem/MPC Models/MPC Model with Spacing Control ==
  Sample time : Inport
  Transport lag : Inport  Port=2
  Longitudinal velocity : Inport  Port=3
  Ag : Inport  Port=4
  Bg : Inport  Port=5
  Cg : Inport  Port=6
  Adaptive Model with Spacing Control : MATLAB Function  TreatAsAtomicUnit=on
  Bus Creator2 : BusCreator  Inputs=8
  DX Constant : Constant  Value=zeros(NumEgoStates+3+4*hasLag,1)  VectorParams1D=off  OutDataTypeStr=pfcsubsystem_data.DataType
  U Constant : Constant  Value=[0;0;InitialLongVel;0]  VectorParams1D=off  OutDataTypeStr=pfcsubsystem_data.DataType
  X Constant : Constant  Value=zeros(NumEgoStates+3+4*hasLag,1)  VectorParams1D=off  OutDataTypeStr=pfcsubsystem_data.DataType
  Y Constant : Constant  Value=[1.4*InitialLongVel+DefaultSpacing;InitialLongVel;0;0]  VectorParams1D=off  OutDataTypeStr=pfcsubsystem_data.DataType
  Model : Outport  VectorParamsAs1DForOutWhenUnconnected=off
  wires:
  Adaptive Model with Spacing Control/4(D) -> Bus Creator2/4  "D"
  X Constant/1 -> Bus Creator2/7  "X"
  Bus Creator2/1 -> Model/1
  Sample time/1 -> Adaptive Model with Spacing Control/1(Ts)
  Adaptive Model with Spacing Control/1(A) -> Bus Creator2/1  "A"
  DX Constant/1 -> Bus Creator2/8  "DX"
  Adaptive Model with Spacing Control/2(B) -> Bus Creator2/2  "B"
  Adaptive Model with Spacing Control/3(C) -> Bus Creator2/3  "C"
  Longitudinal velocity/1 -> Adaptive Model with Spacing Control/2(Vx)
  Y Constant/1 -> Bus Creator2/6  "Y"
  U Constant/1 -> Bus Creator2/5  "U"
  Ag/1 -> Adaptive Model with Spacing Control/3(Ag)
  Bg/1 -> Adaptive Model with Spacing Control/4(Bg)
  Cg/1 -> Adaptive Model with Spacing Control/5(Cg)
  Transport lag/1 -> Adaptive Model with Spacing Control/6(lag)

== system mpc_pathFollowingMod/PFC subsystem/Vehicle Models/Vehicle external model ==
  Vehicle dynamics matrix A : Inport
  Vehicle dynamics matrix B : Inport  Port=2
  Vehicle dynamics matrix C : Inport  Port=3
  DataTypeConversion_A : mpcsigdimcheck_private/DataTypeAutoConversion2D  datatypestr=pfcsubsystem_data.DataType
  DataTypeConversion_B : mpcsigdimcheck_private/DataTypeAutoConversion2D  datatypestr=pfcsubsystem_data.DataType
  DataTypeConversion_C : mpcsigdimcheck_private/DataTypeAutoConversion2D  datatypestr=pfcsubsystem_data.DataType
  Signal Specification A : SignalSpecification
  Signal Specification B : SignalSpecification
  Signal Specification C : SignalSpecification
  A : Outport  VectorParamsAs1DForOutWhenUnconnected=off
  B : Outport  Port=2  VectorParamsAs1DForOutWhenUnconnected=off
  C : Outport  Port=3  VectorParamsAs1DForOutWhenUnconnected=off
  wires:
  Signal Specification B/1 -> B/1
  Signal Specification C/1 -> C/1
  DataTypeConversion_C/1 -> Signal Specification C/1
  Signal Specification A/1 -> A/1
  Vehicle dynamics matrix A/1 -> DataTypeConversion_A/1
  Vehicle dynamics matrix C/1 -> DataTypeConversion_C/1
  DataTypeConversion_A/1 -> Signal Specification A/1
  Vehicle dynamics matrix B/1 -> DataTypeConversion_B/1
  DataTypeConversion_B/1 -> Signal Specification B/1

== system mpc_pathFollowingMod/PFC subsystem/Vehicle Models/Vehicle parametric model ==
  Vx : Inport
  Vehicle combined dynamics : Subsystem
  Vehicle lateral dynamics : Subsystem
  Vehicle longitudinal dynamics : Subsystem
  A : Outport  VectorParamsAs1DForOutWhenUnconnected=off
  B : Outport  Port=2  VectorParamsAs1DForOutWhenUnconnected=off
  C : Outport  Port=3  VectorParamsAs1DForOutWhenUnconnected=off
  wires:
  Vehicle combined dynamics/3(C) -> C/1
  Vehicle combined dynamics/1(A) -> A/1
  Vehicle combined dynamics/2(B) -> B/1
  Vehicle lateral dynamics/1(Am) -> Vehicle combined dynamics/4(A2)
  Vehicle lateral dynamics/2(Bm) -> Vehicle combined dynamics/5(B2)
  Vehicle lateral dynamics/3(Cm) -> Vehicle combined dynamics/6(C2)
  Vehicle longitudinal dynamics/1(An) -> Vehicle combined dynamics/1(A1)
  Vehicle longitudinal dynamics/2(Bn) -> Vehicle combined dynamics/2(B1)
  Vehicle longitudinal dynamics/3(Cn) -> Vehicle combined dynamics/3(C1)
  Vx/1 -> Vehicle lateral dynamics/1(Vx)

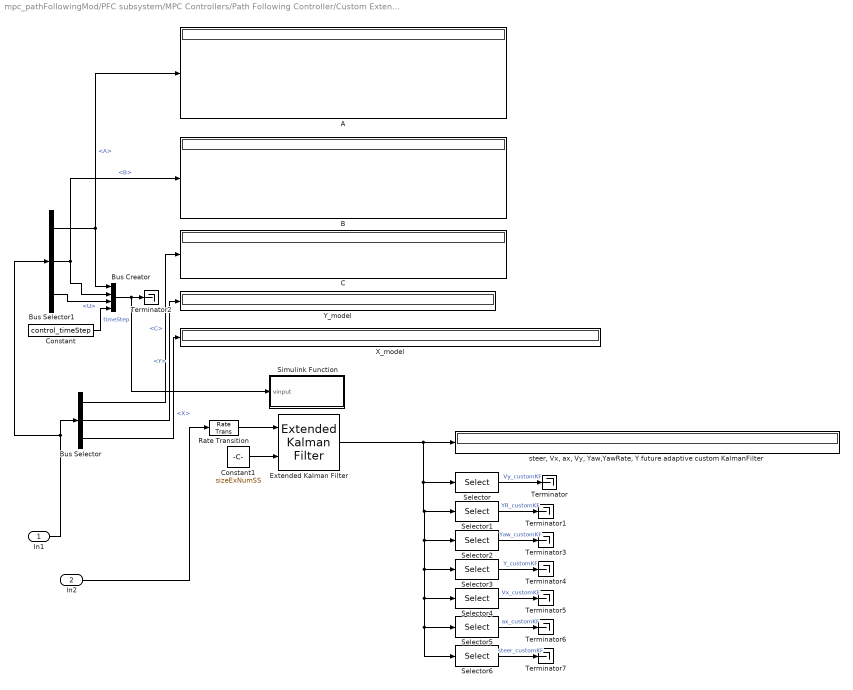
== system mpc_pathFollowingMod/PFC subsystem/MPC Controllers/Path Following Controller/Custom Extented Kalman filter ==
  In1 : Inport
  In2 : Inport  Port=2
  A : Display
  B : Display
  Bus Creator : BusCreator  Inputs=4
  Bus Selector : BusSelector  OutputSignals=C,Y,X
  Bus Selector1 : BusSelector  OutputSignals=A,B,U
  C : Display
  Constant : Constant  Value=control_timeStep
  Constant1 : Constant  Value=sizeExNumSS
  Extended Kalman Filter : sharedTrackingLibrary/Extended Kalman Filter  StateTransitionFcn=statefcn_sl  HasStateTransitionJacobianFcn=off  HasAdditiveProcessNoise=Additive  ProcessNoise=eye(6+sizeExNumSS)*0.1  HasTimeVaryingProcessNoise=off  HasStateTransitionFcnExtraArgument=0  InitialState=state_init.Plant  InitialStateCovariance=eye(6+sizeExNumSS)*0.1  MeasurementFcn1=MeasurementFcn_xVelYPosYaw  HasMeasurementJacobianFcn1=off  HasMeasurementEnablePort1=off  HasAdditiveMeasurementNoise1=Additive  MeasurementNoise1=eye(4)*0.01  HasTimeVaryingMeasurementNoise1=off  HasMeasurementFcnExtraArgument1=1  HasMeasurementWrapping1=off  MeasurementFcn2=myMeasurementFcn  HasMeasurementJacobianFcn2=off  HasMeasurementEnablePort2=off  HasAdditiveMeasurementNoise2=Additive  MeasurementNoise2=1  HasTimeVaryingMeasurementNoise2=off  HasMeasurementFcnExtraArgument2=0  HasMeasurementWrapping2=off  MeasurementFcn3=myMeasurementFcn  HasMeasurementJacobianFcn3=off  HasMeasurementEnablePort3=off  HasAdditiveMeasurementNoise3=Additive  MeasurementNoise3=1  HasTimeVaryingMeasurementNoise3=off  HasMeasurementFcnExtraArgument3=0  HasMeasurementWrapping3=off  MeasurementFcn4=myMeasurementFcn  HasMeasurementJacobianFcn4=off  HasMeasurementEnablePort4=off  HasAdditiveMeasurementNoise4=Additive  MeasurementNoise4=1  HasTimeVaryingMeasurementNoise4=off  HasMeasurementFcnExtraArgument4=0  HasMeasurementWrapping4=off  MeasurementFcn5=myMeasurementFcn  HasMeasurementJacobianFcn5=off  HasMeasurementEnablePort5=off  HasAdditiveMeasurementNoise5=Additive  MeasurementNoise5=1  HasTimeVaryingMeasurementNoise5=off  HasMeasurementFcnExtraArgument5=0  HasMeasurementWrapping5=off  EnableMultirate=off  StateTransitionFcnSampleTime=1  MeasurementFcn1SampleTime=1  MeasurementFcn2SampleTime=1  MeasurementFcn3SampleTime=1  MeasurementFcn4SampleTime=1  MeasurementFcn5SampleTime=1  UseCurrentEstimator=on  OutputStateCovariance=off  DataType=double  SampleTime=control_timeStep  NumberOfMeasurements=1
  Rate Transition : RateTransition  OutPortSampleTime=control_timeStep
  Selector : Selector  InputPortWidth=6+sizeExNumSS  IndexOptions=Index vector (dialog)  Indices=3+sizeExNumSS  OutputSizes=1
  Selector1 : Selector  InputPortWidth=6+sizeExNumSS  IndexOptions=Index vector (dialog)  Indices=5+sizeExNumSS  OutputSizes=1
  Selector2 : Selector  InputPortWidth=6+sizeExNumSS  IndexOptions=Index vector (dialog)  Indices=4+sizeExNumSS  OutputSizes=1
  Selector3 : Selector  InputPortWidth=6+sizeExNumSS  IndexOptions=Index vector (dialog)  Indices=6+sizeExNumSS  OutputSizes=1
  Selector4 : Selector  InputPortWidth=6+sizeExNumSS  IndexOptions=Index vector (dialog)  Indices=1+sizeExNumSS  OutputSizes=1
  Selector5 : Selector  InputPortWidth=6+sizeExNumSS  IndexOptions=Index vector (dialog)  Indices=2+sizeExNumSS  OutputSizes=1
  Selector6 : Selector  InputPortWidth=6+sizeExNumSS  IndexOptions=Index vector (dialog)  Indices=1  OutputSizes=1
  Simulink Function : Subsystem  TreatAsAtomicUnit=on
  Terminator{,1..7} (8 alike) : Terminator
  X_model : Display
  Y_model : Display
  "steer, Vx, ax, Vy, Yaw,YawRate, Y future adaptive custom KalmanFilter" : Display
  wires:
  Bus Creator/1 -> Simulink Function/1(vinput), Terminator2/1
  Bus Selector/3 -> X_model/1  "<X>"
  Bus Selector1/1 -> Bus Creator/1, A/1  "<A>"
  Rate Transition/1 -> Extended Kalman Filter/1
  Constant/1 -> Bus Creator/4  "timeStep"
  Bus Selector/2 -> Y_model/1  "<Y>"
  Bus Selector1/3 -> Bus Creator/3  "<U>"
  Bus Selector/1 -> C/1  "<C>"
  Bus Selector1/2 -> Bus Creator/2, B/1  "<B>"
  In1/1 -> Bus Selector1/1, Bus Selector/1
  In2/1 -> Rate Transition/1
  Constant1/1 -> Extended Kalman Filter/2
  Selector/1 -> Terminator/1  "Vy_customKF"
  Selector1/1 -> Terminator1/1  "YR_customKF"
  Selector2/1 -> Terminator3/1  "Yaw_customKF"
  Selector3/1 -> Terminator4/1  "Y_customKF"
  Selector4/1 -> Terminator5/1  "Vx_customKF"
  Extended Kalman Filter/1 -> Selector6/1, Selector5/1, Selector4/1, Selector3/1, Selector2/1, Selector1/1, Selector/1, "steer, Vx, ax, Vy, Yaw,YawRate, Y future adaptive custom KalmanFilter"/1
  Selector5/1 -> Terminator6/1  "ax_customKF"
  Selector6/1 -> Terminator7/1  "steer_customKF"

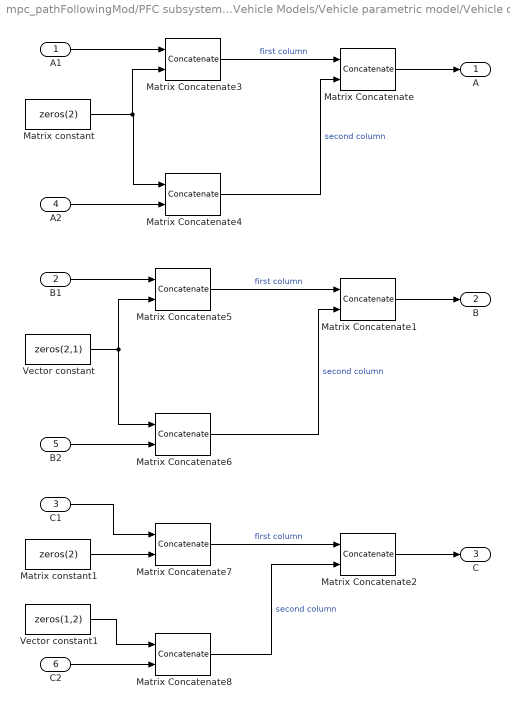
== system mpc_pathFollowingMod/PFC subsystem/Vehicle Models/Vehicle parametric model/Vehicle combined dynamics ==
  A1 : Inport
  B1 : Inport  Port=2
  C1 : Inport  Port=3
  A2 : Inport  Port=4
  B2 : Inport  Port=5
  C2 : Inport  Port=6
  Matrix Concatenate : Concatenate  Mode=Multidimensional array  ConcatenateDimension=2
  Matrix Concatenate1 : Concatenate  Mode=Multidimensional array  ConcatenateDimension=2
  Matrix Concatenate2 : Concatenate  Mode=Multidimensional array  ConcatenateDimension=2
  Matrix Concatenate{3..8} (6 alike) : Concatenate  Mode=Multidimensional array
  Matrix constant : Constant  Value=zeros(2)  VectorParams1D=off  OutDataTypeStr=pfcsubsystem_data.DataType
  Matrix constant1 : Constant  Value=zeros(2)  VectorParams1D=off  OutDataTypeStr=pfcsubsystem_data.DataType
  Vector constant : Constant  Value=zeros(2,1)  VectorParams1D=off  OutDataTypeStr=pfcsubsystem_data.DataType
  Vector constant1 : Constant  Value=zeros(1,2)  VectorParams1D=off  OutDataTypeStr=pfcsubsystem_data.DataType
  A : Outport  VectorParamsAs1DForOutWhenUnconnected=off
  B : Outport  Port=2  VectorParamsAs1DForOutWhenUnconnected=off
  C : Outport  Port=3  VectorParamsAs1DForOutWhenUnconnected=off
  wires:
  Vector constant/1 -> Matrix Concatenate6/1, Matrix Concatenate5/2
  C1/1 -> Matrix Concatenate7/1
  Matrix Concatenate6/1 -> Matrix Concatenate1/2  "second column"
  Matrix Concatenate4/1 -> Matrix Concatenate/2  "second column"
  B1/1 -> Matrix Concatenate5/1
  Matrix Concatenate1/1 -> B/1
  Vector constant1/1 -> Matrix Concatenate8/1
  Matrix Concatenate/1 -> A/1
  Matrix constant/1 -> Matrix Concatenate4/1, Matrix Concatenate3/2
  Matrix Concatenate2/1 -> C/1
  Matrix constant1/1 -> Matrix Concatenate7/2
  Matrix Concatenate8/1 -> Matrix Concatenate2/2  "second column"
  Matrix Concatenate7/1 -> Matrix Concatenate2/1  "first column"
  C2/1 -> Matrix Concatenate8/2
  B2/1 -> Matrix Concatenate6/2
  A2/1 -> Matrix Concatenate4/2
  Matrix Concatenate3/1 -> Matrix Concatenate/1  "first column"
  A1/1 -> Matrix Concatenate3/1
  Matrix Concatenate5/1 -> Matrix Concatenate1/1  "first column"

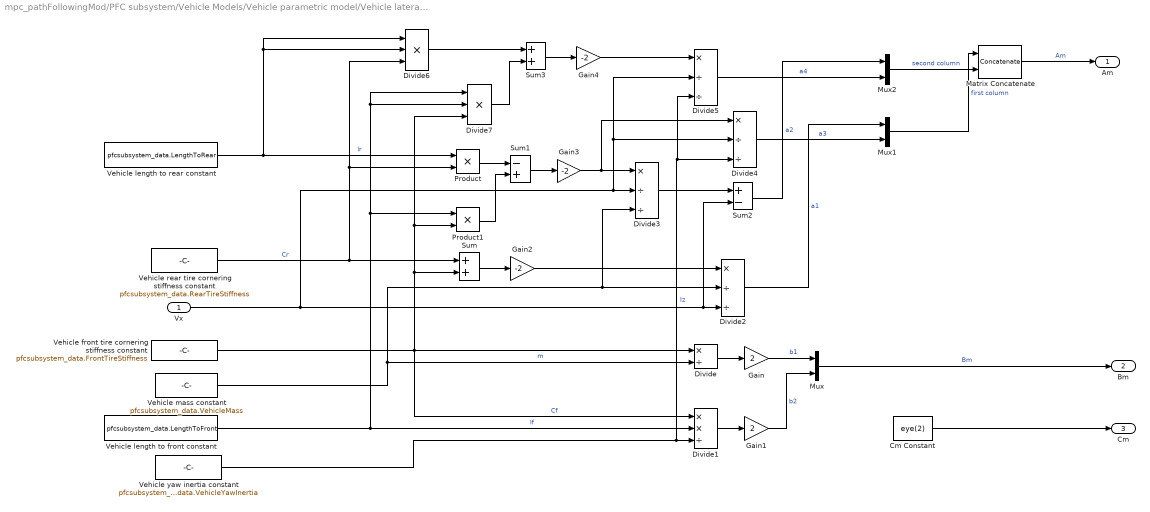
== system mpc_pathFollowingMod/PFC subsystem/Vehicle Models/Vehicle parametric model/Vehicle lateral dynamics ==
  Vx : Inport
  Cm Constant : Constant  Value=eye(2)  OutDataTypeStr=pfcsubsystem_data.DataType
  Divide : Product  Inputs=*/
  Divide1 : Product  Inputs=**/
  Divide{2..5} (4 alike) : Product  Inputs=*//
  Divide6 : Product  Inputs=***
  Divide7 : Product  Inputs=***
  Gain : Gain  Gain=2
  Gain1 : Gain  Gain=2
  Gain2 : Gain  Gain=-2
  Gain3 : Gain  Gain=-2
  Gain4 : Gain  Gain=-2
  Matrix Concatenate : Concatenate  Mode=Multidimensional array  ConcatenateDimension=2
  Mux : Mux  Inputs=[1 1]
  Mux1 : Mux  Inputs=[1 1]
  Mux2 : Mux  Inputs=[1 1]
  Product : Product
  Product1 : Product
  Sum : Sum
  Sum1 : Sum  Inputs=-+
  Sum2 : Sum  Inputs=+-
  Sum3 : Sum
  Vehicle front tire cornering stiffness constant : Constant  Value=pfcsubsystem_data.FrontTireStiffness  OutDataTypeStr=pfcsubsystem_data.DataType
  Vehicle length to front constant : Constant  Value=pfcsubsystem_data.LengthToFront  OutDataTypeStr=pfcsubsystem_data.DataType
  Vehicle length to rear constant : Constant  Value=pfcsubsystem_data.LengthToRear  OutDataTypeStr=pfcsubsystem_data.DataType
  Vehicle mass constant : Constant  Value=pfcsubsystem_data.VehicleMass  OutDataTypeStr=pfcsubsystem_data.DataType
  Vehicle rear tire cornering stiffness constant : Constant  Value=pfcsubsystem_data.RearTireStiffness  OutDataTypeStr=pfcsubsystem_data.DataType
  Vehicle yaw inertia constant : Constant  Value=pfcsubsystem_data.VehicleYawInertia  OutDataTypeStr=pfcsubsystem_data.DataType
  Am : Outport  VectorParamsAs1DForOutWhenUnconnected=off
  Bm : Outport  Port=2  VectorParamsAs1DForOutWhenUnconnected=off
  Cm : Outport  Port=3  VectorParamsAs1DForOutWhenUnconnected=off
  wires:
  Divide5/1 -> Mux2/2  "a4"
  Vehicle length to front constant/1 -> Divide7/1, Divide7/2, Product1/1, Divide1/2  "lf"
  Mux2/1 -> Matrix Concatenate/2  "second column"
  Product1/1 -> Sum1/2
  Vehicle front tire cornering stiffness constant/1 -> Divide1/1, Divide/1, Divide7/3, Product1/2, Sum/2  "Cf"
  Vehicle yaw inertia constant/1 -> Divide5/3, Divide4/3, Divide1/3  "Iz"
  Vehicle mass constant/1 -> Divide/2, Divide3/3, Divide2/2  "m"
  Gain4/1 -> Divide5/1
  Vehicle length to rear constant/1 -> Divide6/2, Divide6/1, Product/1  "lr"
  Vehicle rear tire cornering stiffness constant/1 -> Divide6/3, Product/2, Sum/1  "Cr"
  Sum2/1 -> Mux2/1  "a2"
  Vx/1 -> Divide3/2, Divide5/2, Divide4/2, Sum2/2, Divide2/3
  Gain/1 -> Mux/1  "b1"
  Divide2/1 -> Mux1/1  "a1"
  Product/1 -> Sum1/1
  Mux/1 -> Bm/1  "Bm"
  Divide4/1 -> Mux1/2  "a3"
  Divide7/1 -> Sum3/2
  Matrix Concatenate/1 -> Am/1  "Am"
  Sum3/1 -> Gain4/1
  Gain3/1 -> Divide3/1, Divide4/1
  Sum1/1 -> Gain3/1
  Mux1/1 -> Matrix Concatenate/1  "first column"
  Sum/1 -> Gain2/1
  Divide3/1 -> Sum2/1
  Gain1/1 -> Mux/2  "b2"
  Divide/1 -> Gain/1
  Divide1/1 -> Gain1/1
  Cm Constant/1 -> Cm/1
  Gain2/1 -> Divide2/1
  Divide6/1 -> Sum3/1

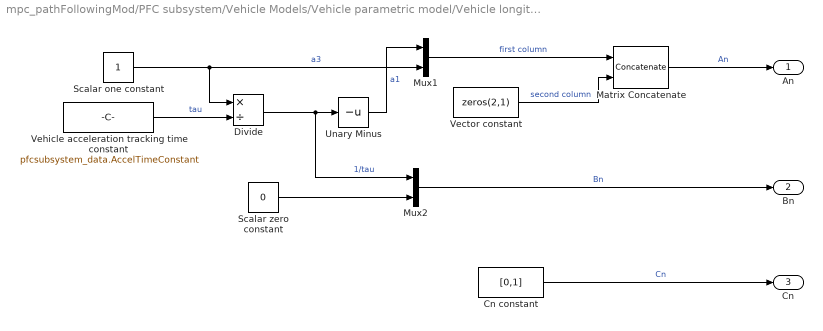
== system mpc_pathFollowingMod/PFC subsystem/Vehicle Models/Vehicle parametric model/Vehicle longitudinal dynamics ==
  Cn constant : Constant  Value=[0,1]  VectorParams1D=off  OutDataTypeStr=pfcsubsystem_data.DataType
  Divide : Product  Inputs=*/
  Matrix Concatenate : Concatenate  Mode=Multidimensional array  ConcatenateDimension=2
  Mux1 : Mux  Inputs=[1 1]
  Mux2 : Mux  Inputs=[1 1]
  Scalar one constant : Constant  OutDataTypeStr=pfcsubsystem_data.DataType
  Scalar zero constant : Constant  Value=0  OutDataTypeStr=pfcsubsystem_data.DataType
  Unary Minus : UnaryMinus
  Vector constant : Constant  Value=zeros(2,1)  VectorParams1D=off  OutDataTypeStr=pfcsubsystem_data.DataType
  Vehicle acceleration tracking time constant : Constant  Value=pfcsubsystem_data.AccelTimeConstant  OutDataTypeStr=pfcsubsystem_data.DataType
  An : Outport  VectorParamsAs1DForOutWhenUnconnected=off
  Bn : Outport  Port=2  VectorParamsAs1DForOutWhenUnconnected=off
  Cn : Outport  Port=3  VectorParamsAs1DForOutWhenUnconnected=off
  wires:
  Vehicle acceleration tracking time constant/1 -> Divide/2  "tau"
  Divide/1 -> Mux2/1, Unary Minus/1  "1/tau"
  Vector constant/1 -> Matrix Concatenate/2  "second column"
  Matrix Concatenate/1 -> An/1  "An"
  Cn constant/1 -> Cn/1  "Cn"
  Unary Minus/1 -> Mux1/1  "a1"
  Scalar one constant/1 -> Mux1/2, Divide/1  "a3"
  Mux2/1 -> Bn/1  "Bn"
  Scalar zero constant/1 -> Mux2/2
  Mux1/1 -> Matrix Concatenate/1  "first column"

== system mpc_pathFollowingMod/PFC subsystem/MPC Controllers/Path Following Controller/Custom Extented Kalman filter/Simulink Function ==
  vinput : Inport
  statefcn_sl : TriggerPort  TriggerType=function-call  IsSimulinkFunction=on  FunctionName=statefcn_sl  FunctionVisibility=scoped  VariantControl=(inherit)
  Bus Selector : BusSelector  OutputSignals=A,B,U,timeStep
  MATLAB Function : MATLAB Function  TreatAsAtomicUnit=on
  u : ArgIn  DisableCoverage=on  PortDimensions=[6+sizeExNumSS, 1]  ArgumentName=u
  y : ArgOut  DisableCoverage=on  PortDimensions=[6+sizeExNumSS, 1]  ArgumentName=y
  wires:
  u/1 -> MATLAB Function/1(x)
  MATLAB Function/1(y) -> y/1
  vinput/1 -> Bus Selector/1
  Bus Selector/1 -> MATLAB Function/2(A)  "<A>"
  Bus Selector/2 -> MATLAB Function/3(B)  "<B>"
  Bus Selector/3 -> MATLAB Function/4(u)  "<U>"
  Bus Selector/4 -> MATLAB Function/5(timeStep)  "<timeStep>"

== matlab function mpc_pathFollowingMod/PFC subsystem/MPC Controllers/Path Following Controller/Custom Extented Kalman filter/Simulink Function/MATLAB Function ==
  data: x input; A input; B input; u input; y output; timeStep input
function y = fcn(x, A, B, u, timeStep)
y = StateFcn_bicycle(x, A, B, u, timeStep);

== matlab function mpc_pathFollowingMod/MATLAB Function2 ==
  data: u input; y output; offset input
function y = fcn(u, offset)
% u: x y yaw_deg z pitch 

y = u(1, :);
rotm = eul2rotm(deg2rad([u(1, 3), u(1, 5), 0]), "ZYX");
offset_3d = rotm * [offset; 0; 0];

y([1, 2, 4]) = u(1, [1, 2, 4]) + offset_3d';

== matlab function mpc_pathFollowingMod/PFC subsystem/MPC Models/MPC Model/Adaptive Model ==
  data: Ts input; A output; Vx input; Ag input; Bg input; Cg input; lag input; B output; C output; D output
function [A,B,C,D] = getAdaptiveMPCModel(Ts,Vx, Ag, Bg, Cg, lag)
% Get discrete state-space model for Adaptive MPC with sample time Ts.
% Called by the 'Path Following Control System' Block.

% Inputs:
%   Ts:               mask variable for sample time
%   Vx:               mask inport for longitudinal velocity
%   Ag,Bg,Cg:         continuous or discrete vehicle model with sample time Ts
% Outputs:
%   A,B,C,D:          discrete time model for adaptive MPC

%   Author: Meng Xia, Rong Chen
%   Copyright 2017-2018 The MathWorks, Inc.

% Discrete MPC model
[A,B,C,D] = pfcblock_utilGetDTModelHasLagForMPCNoSpacingCtrl(Ts,Vx,Ag,Bg,Cg,lag);

== matlab function mpc_pathFollowingMod/PFC subsystem/MPC Models/MPC Model with Spacing Control/Adaptive Model with Spacing Control ==
  data: Ts input; A output; Vx input; Ag input; Bg input; Cg input; lag input; B output; C output; D output
function [A,B,C,D] = getAdaptiveMPCModel(Ts,Vx, Ag, Bg, Cg, lag)
% Get discrete state-space model for Adaptive MPC with sample time Ts.
% Called by the 'Path Following Control System' Block.

% Inputs:
%   Ts:               mask variable for sample time
%   Vx:               mask inport for longitudinal velocity
%   Ag,Bg,Cg:         continuous or discrete vehicle model with sample time Ts
% Outputs:
%   A,B,C,D:          discrete time model for adaptive MPC

%   Author: Meng Xia, Rong Chen
%   Copyright 2017-2018 The MathWorks, Inc.

% Discrete MPC model
[A,B,C,D] = pfcblock_utilGetDTModelHasLagForMPCHasSpacingCtrl(Ts,Vx,Ag,Bg,Cg,lag);

== matlab function mpc_pathFollowingMod/MATLAB Function1 ==
  data: u input; y output; offset input
function y = fcn(u, offset)
% u: x y yaw_deg z pitch 

y = u;
rotm = eul2rotm(deg2rad([u(3), u(5), 0]), "ZYX");
offset_3d = rotm * [offset; 0; 0];

y([1, 2, 4]) = u([1, 2, 4]) + offset_3d';
